simulink model "Controller"  (R2012b)
settings: Solver=FixedStepDiscrete  StartTime=0.0  StopTime=10.0  FixedStep=0.1  RelTol=1e-3
settings Model: Creator=Kerianne  LastModifiedBy=Kerianne
settings DataIOCC: SaveFormat=Structure
settings OptimizationCC: InlineParams=on

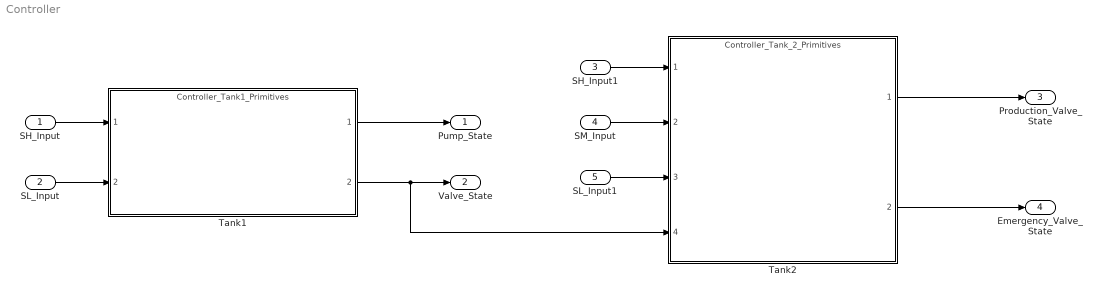
== system Controller ==
  SH_Input : Inport  OutDataTypeStr=double
  SL_Input : Inport  Port=2  OutDataTypeStr=double
  SH_Input1 : Inport  Port=3  OutDataTypeStr=double
  SM_Input : Inport  Port=4  OutDataTypeStr=double
  SL_Input1 : Inport  Port=5  OutDataTypeStr=double
  Tank1 : ModelReference  ModelNameDialog=Controller_Tank1_Primitives  SimulationMode=Normal  ModelReferenceVersion=1.35  CopyOfModelName=Controller_Tank1_Primitives  DefaultDataLogging=on
  Tank2 : ModelReference  ModelNameDialog=Controller_Tank_2_Primitives  SimulationMode=Normal  ModelReferenceVersion=1.32  CopyOfModelName=Controller_Tank_2_Primitives  DefaultDataLogging=on
  Pump_State : Outport  OutDataTypeStr=double
  Valve_State : Outport  Port=2  OutDataTypeStr=double
  Production_Valve_State : Outport  Port=3  OutDataTypeStr=double
  Emergency_Valve_State : Outport  Port=4  OutDataTypeStr=double
  wires:
  SH_Input/1 -> Tank1/1
  SL_Input/1 -> Tank1/2
  SH_Input1/1 -> Tank2/1
  SL_Input1/1 -> Tank2/3
  SM_Input/1 -> Tank2/2
  Tank2/2 -> Emergency_Valve_State/1
  Tank2/1 -> Production_Valve_State/1
  Tank1/1 -> Pump_State/1
  Tank1/2 -> Tank2/4, Valve_State/1
